simulink library "AEMS_Standard_Library"  (R2016b)
settings: Solver=ode45  StartTime=0.0  StopTime=10.0  RelTol=1e-3
undefined symbols (not defined in the file or in its folder): BkPY, carto, Cbx_extegr, Cbx_lpegrsys, Cbx_portegr, Cnx_bnk_nr_conf, Cnx_cyl_nr_conf, ConfigManagement, configuration_management, Cxx_dcm_io_tmr_end_xxxx, Cxx_dcm_rt_tmr_end, Cxx_DID_xxxx_IO_max, Cxx_DID_xxxx_IO_min, Cxx_egrhsofs, Cxx_vmaniegi, DEM_DEBOUNCE_FREEZE, DEM_DTR_CTL_INVISIBLE, DEM_DTR_CTL_NORMAL, Dem_DtrId2_XXX, Dem_DtrId3_XXX, Dem_DtrId4_XXX, Dem_DtrId5_XXX, Dem_DtrId6_XXX, Dem_DtrId7_XXX, Dem_DtrId8_XXX, Dem_DtrId9_XXX, Dem_DtrId_XXX, Dem_EnableConditionId2_XXX, Dem_EnableConditionId3_XXX, Dem_EnableConditionId4_XXX, Dem_EnableConditionId5_XXX, Dem_EnableConditionId6_XXX, Dem_EnableConditionId7_XXX, Dem_EnableConditionId8_XXX, Dem_EnableConditionId_XXX, Dem_EventId, Dem_EventId2_XXX, Dem_EventId3_XXX, Dem_EventId4_XXX, Dem_EventId5_XXX, Dem_EventId6_XXX, Dem_EventId7_XXX, Dem_EventId8_XXX, Dem_EventId9_XXX, Dem_EventId_Device_Faulttype, Dem_EventId_XXX, DEM_IUMPR_GENERAL_DENOMINATOR, DEM_OPCYC_IGNITION, Dem_RatioId2_XXX, Dem_RatioId3_XXX, Dem_RatioId4_XXX, Dem_RatioId5_XXX, Dem_RatioId6_XXX, Dem_RatioId7_XXX, Dem_RatioId8_XXX, Dem_RatioId_XXX, Dem_StorageConditionId2_XXX, Dem_StorageConditionId3_XXX, Dem_StorageConditionId4_XXX, Dem_StorageConditionId5_XXX ... (+65)
libraries: AEMS_Standard_Library x477, simulink x2
(part 18 of 39)

== system AEMS_Standard_Library/SPECIFIC/AEMS_AIR_BALANCE ==
  rpm : Inport  OutDataTypeStr=single  PortDimensions=1  Interpolate=off
  vcyl : Inport  Port=2  OutDataTypeStr=single  PortDimensions=1  Interpolate=off
  egclrt : Inport  Port=3  OutDataTypeStr=single  PortDimensions=1  Interpolate=off
  tanmnp : Inport  Port=4  OutDataTypeStr=single  PortDimensions=1  Interpolate=off
  fqselgo : Inport  Port=5  OutDataTypeStr=boolean  PortDimensions=1  Interpolate=off
  pargeqd : Inport  Port=6  OutDataTypeStr=single  PortDimensions=1  Interpolate=off
  qegrve : Inport  Port=7  OutDataTypeStr=single  PortDimensions=1  Interpolate=off
  ppamb : Inport  Port=8  OutDataTypeStr=single  PortDimensions=1  Interpolate=off
  qtrm : Inport  Port=9  OutDataTypeStr=single  PortDimensions=1  Interpolate=off
  qegrth : Inport  Port=10  OutDataTypeStr=single  PortDimensions=1  Interpolate=off
  fafmlmsta : Inport  Port=11  OutDataTypeStr=boolean  PortDimensions=1  Interpolate=off
  qcylegr_p : Inport  Port=12  OutDataTypeStr=single  PortDimensions=1  Interpolate=off
  vmani : Inport  Port=13  OutDataTypeStr=single  PortDimensions=1  Interpolate=off
  fair_egrv : Inport  Port=14  OutDataTypeStr=boolean  Interpolate=off
  MWI_Cyl_Charge_Mass_Air_N : Subsystem  Description=|
      | Air,EGR or (Air + EGR) mass of cylinder is calculated.                
      | Qcyl(kg/s)                                                            
      | = mamani(kg/1 cycle 1cylinder) * rpm * Nref(number of cylinder/2) * 60
  MWI_Mani_Charge_Mass_Air_EGR : Subsystem  Description=Air,EGR or (air+EGR) mass of correcter is calculated.
  MWI_Manifold_Pressure_N : Subsystem  Description=Pressure of correcter is calculated by the state equation.
  Unit Delay4 : UnitDelay  SampleTime=-1
      settings: AttributesFormatString=<initial=%<InitialCondition>>
  Unit Delay5 : UnitDelay  SampleTime=-1
      settings: AttributesFormatString=<initial=%<InitialCondition>>
  Unit Delay6 : UnitDelay  SampleTime=-1
      settings: AttributesFormatString=<initial=%<InitialCondition>>
  mamani : Outport
  airmani : Outport  Port=2
  macyllj : Outport  Port=3
  qcylall : Outport  Port=4
  qcylegr : Outport  Port=5
  qcyl : Outport  Port=6
  pmani : Outport  Port=7
  egrmani : Outport  Port=8
  egclrt_p : Outport  Port=9
  wires:
  vmani/1 -> MWI_Manifold_Pressure_N/1(vmani), MWI_Cyl_Charge_Mass_Air_N/5(vmani), MWI_Mani_Charge_Mass_Air_EGR/9(vmani)  "vmani"
  MWI_Cyl_Charge_Mass_Air_N/5(egclrt_p) -> egclrt_p/1
  qcylegr_p/1 -> MWI_Cyl_Charge_Mass_Air_N/4(qcylegr_p)  "qcylegr_p"
  fafmlmsta/1 -> MWI_Mani_Charge_Mass_Air_EGR/8(fafmlmsta)  "fafmlmsta"
  qegrth/1 -> MWI_Mani_Charge_Mass_Air_EGR/7(qegrth)  "qegrth"
  qtrm/1 -> MWI_Mani_Charge_Mass_Air_EGR/6(qtrm)  "qtrm"
  ppamb/1 -> MWI_Mani_Charge_Mass_Air_EGR/5(ppamb)  "ppamb"
  qegrve/1 -> MWI_Mani_Charge_Mass_Air_EGR/4(qegrve)  "qegrve"
  pargeqd/1 -> MWI_Mani_Charge_Mass_Air_EGR/3(pargeqd)  "pargeqd"
  fqselgo/1 -> MWI_Mani_Charge_Mass_Air_EGR/2(fqselgo)  "fqselgo"
  tanmnp/1 -> MWI_Manifold_Pressure_N/2(tanmnp), MWI_Mani_Charge_Mass_Air_EGR/1(tanmnp)  "tanmnp"
  egclrt/1 -> MWI_Cyl_Charge_Mass_Air_N/3(egclrt)  "egclrt"
  vcyl/1 -> MWI_Cyl_Charge_Mass_Air_N/2(vcyl)  "vcyl"
  rpm/1 -> MWI_Cyl_Charge_Mass_Air_N/1(rpm)  "rpm"
  MWI_Mani_Charge_Mass_Air_EGR/2(airmani) -> MWI_Manifold_Pressure_N/3(airmani), airmani/1
  MWI_Cyl_Charge_Mass_Air_N/4(macyllj) -> macyllj/1
  MWI_Manifold_Pressure_N/1(pmani) -> pmani/1
  Unit Delay6/1 -> MWI_Mani_Charge_Mass_Air_EGR/11(qcyl_pudt)  "qcyl_pudt"
  Unit Delay4/1 -> MWI_Mani_Charge_Mass_Air_EGR/12(qcylegr_pudt)  "qcylegr_pudt"
  Unit Delay5/1 -> MWI_Mani_Charge_Mass_Air_EGR/13(qcylall_pudt)  "qcylall_pudt"
  MWI_Mani_Charge_Mass_Air_EGR/3(egrmani) -> egrmani/1, MWI_Manifold_Pressure_N/4(egrmani)
  MWI_Mani_Charge_Mass_Air_EGR/1(mamani) -> MWI_Cyl_Charge_Mass_Air_N/6(mamani), mamani/1
  MWI_Cyl_Charge_Mass_Air_N/3(qcylall) -> qcylall/1, Unit Delay5/1
  MWI_Cyl_Charge_Mass_Air_N/2(qcylegr) -> qcylegr/1, Unit Delay4/1
  MWI_Cyl_Charge_Mass_Air_N/1(qcyl) -> Unit Delay6/1, qcyl/1
  fair_egrv/1 -> MWI_Mani_Charge_Mass_Air_EGR/10(fair_egrv)  "fair_egrv"

== system AEMS_Standard_Library/SPECIFIC/AEMS_AS_PADE ==
  Filter_param : Inport
  Vxx_in : Inport  Port=2
  Vxx_dly_t : Inport  Port=3
  Vbx_dly_init_ena : Inport  Port=4
  A_pade_model : Subsystem
  Saturation : Saturate  UpperLimit=2000  LowerLimit=0  RndMeth=Zero
      settings: AttributesFormatString=<limits=%<UpperLimit>/%<LowerLimit>>
  Vxx_in_dly : Outport
  Vxx_in_fil : Outport  Port=2
  wires:
  A_pade_model/1(Vxx_in_dly) -> Vxx_in_dly/1
  Vxx_in/1 -> A_pade_model/2(Vxx_in)
  Vbx_dly_init_ena/1 -> A_pade_model/4(Vbx_dly_init_ena)
  Vxx_dly_t/1 -> A_pade_model/3(Vxx_dly_t)
  A_pade_model/2(Vxx_in_fil) -> Saturation/1
  Saturation/1 -> Vxx_in_fil/1
  Filter_param/1 -> A_pade_model/1(Filter_param)

== system AEMS_Standard_Library/SPECIFIC/AEMS_AT_EHR ==
  Vxx_ehr_sel_tenv : Inport
  Vxx_ehr_sys_egaf : Inport  Port=2
  Vxx_ehr_cnvt_fac : Inport  Port=3
  Vxx_ehr_ext_exch_ar : Inport  Port=4
  Vxx_ehr_wht : Inport  Port=5
  Vxx_ehr_utp : Inport  Port=6
  Vxx_ehr_cata_temp_dly : Inport  Port=7
  Vxx_ehr_exo_pow : Inport  Port=8
  Vxx_ehr_spc_ex_gas_temp_cpy : Inport  Port=9
  Vxx_ehr_spc_cata_temp_cpy : Inport  Port=10
  Vxx_ehr_samp_t : Inport  Port=11
  A_Enabled_Calculation : Subsystem
  Vxx_ehr_dtp : Outport
  Vxx_ehr_ext_pow_loss : Outport  Port=2
  Vxx_ehr_wht_entr : Outport  Port=3
  Vxx_ehr_ex_gas_entr : Outport  Port=4
  Vxx_ehr_ext_cnvt_entr : Outport  Port=5
  Vxx_ehr_exo_temp_flu : Outport  Port=6
  Vxx_ehr_wht_temp_flu : Outport  Port=7
  Vxx_ehr_ex_gas_temp_flu : Outport  Port=8
  Vxx_ehr_ext_cnvt_temp_flu : Outport  Port=9
  wires:
  Vxx_ehr_sel_tenv/1 -> A_Enabled_Calculation/1(Vxx_ehr_sel_tenv)
  Vxx_ehr_cnvt_fac/1 -> A_Enabled_Calculation/2(Vxx_ehr_cnvt_fac)
  Vxx_ehr_ext_exch_ar/1 -> A_Enabled_Calculation/3(Vxx_ehr_ext_exch_ar)
  Vxx_ehr_samp_t/1 -> A_Enabled_Calculation/4(Vxx_ehr_samp_t)
  Vxx_ehr_utp/1 -> A_Enabled_Calculation/7(Vxx_ehr_utp)
  Vxx_ehr_sys_egaf/1 -> A_Enabled_Calculation/5(Vxx_ehr_sys_egaf)
  Vxx_ehr_spc_ex_gas_temp_cpy/1 -> A_Enabled_Calculation/10(Vxx_ehr_spc_ex_gas_temp_cpy)
  Vxx_ehr_spc_cata_temp_cpy/1 -> A_Enabled_Calculation/11(Vxx_ehr_spc_cata_temp_cpy)
  Vxx_ehr_cata_temp_dly/1 -> A_Enabled_Calculation/8(Vxx_ehr_cata_temp_dly)
  Vxx_ehr_exo_pow/1 -> A_Enabled_Calculation/9(Vxx_ehr_exo_pow)
  Vxx_ehr_wht/1 -> A_Enabled_Calculation/6(Vxx_ehr_wht)
  A_Enabled_Calculation/1(Vxx_ehr_dtp) -> Vxx_ehr_dtp/1
  A_Enabled_Calculation/2(Vxx_ehr_ext_pow_loss) -> Vxx_ehr_ext_pow_loss/1
  A_Enabled_Calculation/3(Vxx_ehr_wht_entr) -> Vxx_ehr_wht_entr/1
  A_Enabled_Calculation/4(Vxx_ehr_ex_gas_entr) -> Vxx_ehr_ex_gas_entr/1
  A_Enabled_Calculation/5(Vxx_ehr_ext_cnvt_entr) -> Vxx_ehr_ext_cnvt_entr/1
  A_Enabled_Calculation/6(Vxx_ehr_exo_temp_flu) -> Vxx_ehr_exo_temp_flu/1
  A_Enabled_Calculation/7(Vxx_ehr_wht_temp_flu) -> Vxx_ehr_wht_temp_flu/1
  A_Enabled_Calculation/8(Vxx_ehr_ex_gas_temp_flu) -> Vxx_ehr_ex_gas_temp_flu/1
  A_Enabled_Calculation/9(Vxx_ehr_ext_cnvt_temp_flu) -> Vxx_ehr_ext_cnvt_temp_flu/1

== system AEMS_Standard_Library/SPECIFIC/AEMS_AT_TUBE ==
  Vxx_tub_utp : Inport
  Vxx_tub_utp_dly : Inport  Port=2
  Vxx_tub_egaf : Inport  Port=3
  Vxx_tub_temp_air : Inport  Port=4
  Vxx_tub_pow_ext : Inport  Port=5
  Vxx_tub_itl_ar : Inport  Port=6
  Vxx_tub_itl_cnvt_fac : Inport  Port=7
  Vxx_tub_ext_ar : Inport  Port=8
  Vxx_tub_ext_cnvt_fac : Inport  Port=9
  Vxx_tub_wht : Inport  Port=10
  Vxx_tub_temp_rd_loss : Inport  Port=11
  Vxx_tub_itl_gas_wht_cor : Inport  Port=12
  Vxx_tub_cal_cpy : Inport  Port=13
  Vxx_tub_gas_cal_cpy : Inport  Port=14
  Vxx_tub_utp_gas_wht_cor : Inport  Port=15
  Vxx_tub_samp_t : Inport  Port=16
  Vxx_tub_temp_esti_dly : Inport  Port=17
  Vxx_tub_ex_gas_dtp_esti_dly : Inport  Port=18
  A_Thermal_Calculation : Subsystem
  Vxx_tub_ex_gas_dtp_esti : Outport
  Vxx_tub_temp_esti : Outport  Port=2
  Vxx_tub_ex_gas_pow_loss : Outport  Port=3
  Vxx_tub_temp_pow_loss : Outport  Port=4
  Vxx_tub_temp_rd_entr : Outport  Port=5
  Vxx_tub_wht_entr : Outport  Port=6
  Vxx_tub_itl_cnvt_entr : Outport  Port=7
  Vxx_tub_ext_cnvt_entr : Outport  Port=8
  Vxx_tub_entr_tot : Outport  Port=9
  Vxx_tub_ext_cnvt_temp_flu : Outport  Port=10
  Vxx_tub_itl_cnvt_temp_flu : Outport  Port=11
  Vxx_tub_wht_temp_flu : Outport  Port=12
  Vxx_tub_ex_gas_entr : Outport  Port=13
  Vxx_tub_itl_gas_wht_entr : Outport  Port=14
  Vxx_tub_itl_gas_cnvt_entr : Outport  Port=15
  Vxx_tub_gas_entr_tot : Outport  Port=16
  Vxx_tub_gas_temp_flu : Outport  Port=17
  Vxx_tub_gas_wht_temp_flu : Outport  Port=18
  Vxx_tub_gas_itl_cnvt_temp_flu : Outport  Port=19
  Vxx_tub_gas_utp_wht_temp_flu : Outport  Port=20
  Vxx_tub_gas_ext_egy_temp_flu : Outport  Port=21
  wires:
  A_Thermal_Calculation/21(Vxx_tub_gas_ext_egy_temp_flu) -> Vxx_tub_gas_ext_egy_temp_flu/1
  A_Thermal_Calculation/20(Vxx_tub_gas_utp_wht_temp_flu) -> Vxx_tub_gas_utp_wht_temp_flu/1
  A_Thermal_Calculation/19(Vxx_tub_gas_itl_cnvt_temp_flu) -> Vxx_tub_gas_itl_cnvt_temp_flu/1
  A_Thermal_Calculation/18(Vxx_tub_gas_wht_temp_flu) -> Vxx_tub_gas_wht_temp_flu/1
  A_Thermal_Calculation/17(Vxx_tub_gas_temp_flu) -> Vxx_tub_gas_temp_flu/1
  A_Thermal_Calculation/16(Vxx_tub_gas_entr_tot) -> Vxx_tub_gas_entr_tot/1
  A_Thermal_Calculation/15(Vxx_tub_itl_gas_cnvt_entr) -> Vxx_tub_itl_gas_cnvt_entr/1
  A_Thermal_Calculation/14(Vxx_tub_itl_gas_wht_entr) -> Vxx_tub_itl_gas_wht_entr/1
  A_Thermal_Calculation/13(Vxx_tub_ex_gas_entr) -> Vxx_tub_ex_gas_entr/1
  A_Thermal_Calculation/12(Vxx_tub_wht_temp_flu) -> Vxx_tub_wht_temp_flu/1
  A_Thermal_Calculation/11(Vxx_tub_itl_cnvt_temp_flu) -> Vxx_tub_itl_cnvt_temp_flu/1
  A_Thermal_Calculation/10(Vxx_tub_ext_cnvt_temp_flu) -> Vxx_tub_ext_cnvt_temp_flu/1
  A_Thermal_Calculation/9(Vxx_tub_entr_tot) -> Vxx_tub_entr_tot/1
  A_Thermal_Calculation/8(Vxx_tub_ext_cnvt_entr) -> Vxx_tub_ext_cnvt_entr/1
  A_Thermal_Calculation/7(Vxx_tub_itl_cnvt_entr) -> Vxx_tub_itl_cnvt_entr/1
  A_Thermal_Calculation/6(Vxx_tub_wht_entr) -> Vxx_tub_wht_entr/1
  A_Thermal_Calculation/5(Vxx_tub_temp_rd_entr) -> Vxx_tub_temp_rd_entr/1
  A_Thermal_Calculation/4(Vxx_tub_temp_pow_loss) -> Vxx_tub_temp_pow_loss/1
  A_Thermal_Calculation/3(Vxx_tub_ex_gas_pow_loss) -> Vxx_tub_ex_gas_pow_loss/1
  A_Thermal_Calculation/2(Vxx_tub_temp_esti) -> Vxx_tub_temp_esti/1
  A_Thermal_Calculation/1(Vxx_tub_ex_gas_dtp_esti) -> Vxx_tub_ex_gas_dtp_esti/1
  Vxx_tub_ex_gas_dtp_esti_dly/1 -> A_Thermal_Calculation/18(Vxx_tub_ex_gas_dtp_esti_dly)
  Vxx_tub_temp_esti_dly/1 -> A_Thermal_Calculation/17(Vxx_tub_temp_esti_dly)
  Vxx_tub_samp_t/1 -> A_Thermal_Calculation/16(Vxx_tub_samp_t)
  Vxx_tub_utp_gas_wht_cor/1 -> A_Thermal_Calculation/15(Vxx_tub_utp_gas_wht_cor)
  Vxx_tub_gas_cal_cpy/1 -> A_Thermal_Calculation/14(Vxx_tub_gas_cal_cpy)
  Vxx_tub_cal_cpy/1 -> A_Thermal_Calculation/13(Vxx_tub_cal_cpy)
  Vxx_tub_itl_gas_wht_cor/1 -> A_Thermal_Calculation/12(Vxx_tub_itl_gas_wht_cor)
  Vxx_tub_temp_rd_loss/1 -> A_Thermal_Calculation/11(Vxx_tub_temp_rd_loss)
  Vxx_tub_wht/1 -> A_Thermal_Calculation/10(Vxx_tub_wht)
  Vxx_tub_ext_cnvt_fac/1 -> A_Thermal_Calculation/9(Vxx_tub_ext_cnvt_fac)
  Vxx_tub_ext_ar/1 -> A_Thermal_Calculation/8(Vxx_tub_ext_ar)
  Vxx_tub_itl_cnvt_fac/1 -> A_Thermal_Calculation/7(Vxx_tub_itl_cnvt_fac)
  Vxx_tub_itl_ar/1 -> A_Thermal_Calculation/6(Vxx_tub_itl_ar)
  Vxx_tub_pow_ext/1 -> A_Thermal_Calculation/5(Vxx_tub_pow_ext)
  Vxx_tub_temp_air/1 -> A_Thermal_Calculation/4(Vxx_tub_temp_air)
  Vxx_tub_egaf/1 -> A_Thermal_Calculation/3(Vxx_tub_egaf)
  Vxx_tub_utp_dly/1 -> A_Thermal_Calculation/2(Vxx_tub_utp_dly)
  Vxx_tub_utp/1 -> A_Thermal_Calculation/1(Vxx_tub_utp)

== system AEMS_Standard_Library/SPECIFIC/AEMS_BACKUP_FOR_ENGINE_OFF_MONITOR ==
  set : Inport  OutDataTypeStr=boolean
  AND : Logic  OutDataTypeStr=boolean
  AND1 : Logic  Operator=OR  OutDataTypeStr=boolean
  Unit Delay : UnitDelay  SampleTime=-1
      settings: AttributesFormatString=<initial=%<InitialCondition>>
  Unit Delay1 : UnitDelay  SampleTime=-1
      settings: AttributesFormatString=<initial=%<InitialCondition>>
  one : Constant  OutDataTypeStr=boolean
  flag : Outport
  wires:
  Unit Delay/1 -> AND/2
  AND1/1 -> flag/1, Unit Delay/1  "flag"
  set/1 -> AND1/1  "set"
  AND/1 -> AND1/2
  one/1 -> Unit Delay1/1  "one"
  Unit Delay1/1 -> AND/1

== system AEMS_Standard_Library/SPECIFIC/AEMS_BACK_UP ==
  start_flag : Inport
      settings: AttributesFormatString=<tsample=%<sampleTime>>
  vback_up_variable : Inport  Port=2
      settings: AttributesFormatString=<tsample=%<sampleTime>>
  MinMax1 : MinMax  Function=max  Inputs=2  SaturateOnIntegerOverflow=on  InputSameDT=on
  MinMax3 : MinMax  Inputs=2  SaturateOnIntegerOverflow=on  InputSameDT=on
  Switch1 : Switch  Criteria=u2 ~= 0  InputSameDT=on
      settings: AttributesFormatString=Criteria=%<Criteria>
  Switch2 : Switch  Criteria=u2 ~= 0  InputSameDT=on
      settings: AttributesFormatString=Criteria=%<Criteria>
  Switch4 : Switch  Criteria=u2 ~= 0  InputSameDT=on
      settings: AttributesFormatString=Criteria=%<Criteria>
  Unit Delay : UnitDelay  InitialCondition=max_parameter  SampleTime=-1
      settings: AttributesFormatString=<initial=%<InitialCondition>>
  Unit Delay1 : UnitDelay  InitialCondition=min_parameter  SampleTime=-1
      settings: AttributesFormatString=<initial=%<InitialCondition>>
  Unit Delay3 : UnitDelay  SampleTime=-1
      settings: AttributesFormatString=<initial=%<InitialCondition>>
  vend_value : Outport
  vmin_value : Outport  Port=2
  vmax_value : Outport  Port=3
  wires:
  vback_up_variable/1 -> Switch4/1, MinMax3/1, MinMax1/1  "vback_up_variable"
  Switch1/1 -> Unit Delay/1, vmin_value/1  "vmin_value"
  Unit Delay/1 -> MinMax3/2, Switch1/3
  MinMax3/1 -> Switch1/1
  Switch2/1 -> Unit Delay1/1, vmax_value/1  "vmax_value"
  Unit Delay1/1 -> MinMax1/2, Switch2/3
  MinMax1/1 -> Switch2/1
  start_flag/1 -> Switch4/2, Switch1/2, Switch2/2  "start_flag"
  Unit Delay3/1 -> Switch4/3
  Switch4/1 -> Unit Delay3/1, vend_value/1  "vend_value"

== system AEMS_Standard_Library/SPECIFIC/AEMS_BACK_UP_AVE ==
  start_flag : Inport
      settings: AttributesFormatString=<tsample=%<sampleTime>>
  vback_up_variable : Inport  Port=2
      settings: AttributesFormatString=<tsample=%<sampleTime>>
  AEMS_COUNTER : AEMS_Standard_Library/COUNTER/AEMS_COUNTER  Tag=[LIB]  mMAX=2byte
      settings: AttributesFormatString=%<MaskType>\nMax. count range = %<mMAX>
  MinMax1 : MinMax  Function=max  Inputs=2  SaturateOnIntegerOverflow=on  InputSameDT=on
  MinMax2 : MinMax  Function=max  Inputs=2  SaturateOnIntegerOverflow=on  InputSameDT=on
  MinMax3 : MinMax  Inputs=2  SaturateOnIntegerOverflow=on  InputSameDT=on
  MinMax5 : MinMax  Function=max  Inputs=2  SaturateOnIntegerOverflow=on  InputSameDT=on
  MinMax6 : MinMax  Inputs=2  SaturateOnIntegerOverflow=on  InputSameDT=on
  Product1 : Product  Inputs=**  OutDataTypeStr=Inherit: Inherit via back propagation  SaturateOnIntegerOverflow=on  RndMeth=Zero
      settings: AttributesFormatString=SAT = %<SaturateOnIntegerOverflow>
  Product3 : Product  Inputs=*/  OutDataTypeStr=Inherit: Inherit via back propagation  RndMeth=Zero
  Product4 : Product  Inputs=**  OutDataTypeStr=Inherit: Inherit via back propagation  SaturateOnIntegerOverflow=on  RndMeth=Zero
      settings: AttributesFormatString=SAT = %<SaturateOnIntegerOverflow>
  Sum1 : Sum  SaturateOnIntegerOverflow=on  InputSameDT=on  OutDataTypeStr=Inherit: Same as first input
  Switch{1..5} (5 alike) : Switch  Criteria=u2 ~= 0  InputSameDT=on
      settings: AttributesFormatString=Criteria=%<Criteria>
  Unit Delay : UnitDelay  InitialCondition=max_parameter  SampleTime=-1
      settings: AttributesFormatString=<initial=%<InitialCondition>>
  Unit Delay1 : UnitDelay  InitialCondition=min_parameter  SampleTime=-1
      settings: AttributesFormatString=<initial=%<InitialCondition>>
  Unit Delay2 : UnitDelay  SampleTime=-1
      settings: AttributesFormatString=<initial=%<InitialCondition>>
  Unit Delay3 : UnitDelay  SampleTime=-1
      settings: AttributesFormatString=<initial=%<InitialCondition>>
  Unit Delay4 : UnitDelay  SampleTime=-1
      settings: AttributesFormatString=<initial=%<InitialCondition>>
  imm_const1 : Constant  OutDataTypeStr=Inherit: Inherit via back propagation
  imm_const2 : Constant  Value=min_parameter  OutDataTypeStr=Inherit: Inherit via back propagation
  imm_const3 : Constant  Value=0  OutDataTypeStr=boolean
  imm_const5 : Constant  Value=65535  OutDataTypeStr=Inherit: Inherit via back propagation
  imm_const6 : Constant  Value=max_parameter  OutDataTypeStr=Inherit: Inherit via back propagation
  vend_value : Outport
  vmin_value : Outport  Port=2
  vmax_value : Outport  Port=3
  vaverage_value : Outport  Port=4
  wires:
  MinMax1/1 -> Switch2/1
  Unit Delay3/1 -> Switch4/3
  Switch4/1 -> vend_value/1, Unit Delay3/1  "vend_value"
  imm_const2/1 -> Product1/1
  imm_const6/1 -> Product4/1
  imm_const5/1 -> Product4/2, Product1/2  "vmax_count"
  Switch5/1 -> vaverage_value/1, Unit Delay4/1  "vaverage_value"
  Unit Delay4/1 -> Switch5/3
  imm_const3/1 -> AEMS_COUNTER/2  "clear"
  Sum1/1 -> MinMax6/1  "vsum_value"
  Product1/1 -> MinMax5/2
  MinMax6/1 -> MinMax5/1
  MinMax5/1 -> Switch3/1
  Product4/1 -> MinMax6/2
  Product3/1 -> Switch5/1  "average"
  start_flag/1 -> Switch3/2, AEMS_COUNTER/1, Switch5/2, Switch2/2, Switch1/2, Switch4/2
  Switch3/1 -> Unit Delay2/1, Product3/1  "vsum_value"
  imm_const1/1 -> MinMax2/1
  MinMax2/1 -> Product3/2
  Unit Delay2/1 -> Sum1/2, Switch3/3
  AEMS_COUNTER/1 -> MinMax2/2
  vback_up_variable/1 -> MinMax3/1, Sum1/1, MinMax1/1, Switch4/1
  Unit Delay1/1 -> Switch2/3, MinMax1/2
  MinMax3/1 -> Switch1/1
  Unit Delay/1 -> Switch1/3, MinMax3/2
  Switch2/1 -> vmax_value/1, Unit Delay1/1  "vmax_value"
  Switch1/1 -> vmin_value/1, Unit Delay/1  "vmin_value"

== system AEMS_Standard_Library/SPECIFIC/AEMS_DGNDMDPGCUT ==
  note: DGNDMDPGCUT
  mpr : Inport
  dgndmdpc : Inport  Port=2
  kdutydgn : Inport  Port=3
  mxmprp : Inport  Port=4
  AEMS_EDGE_RISING : AEMS_Standard_Library/EDGE/AEMS_EDGE_RISING  Tag=[LIB]  init=false
      settings: AttributesFormatString=|
      | %<MaskType>
      | Initial Value : %<init>
  Product1 : Product  OutDataTypeStr=Inherit: Inherit via back propagation  RndMeth=Zero
  Switch : Switch  Criteria=u2 ~= 0  SaturateOnIntegerOverflow=on  InputSameDT=on
      settings: AttributesFormatString=Criteria=%<Criteria>
  Switch1 : Switch  Criteria=u2 ~= 0  SaturateOnIntegerOverflow=on  InputSameDT=on
      settings: AttributesFormatString=Criteria=%<Criteria>
  Unit Delay3 : UnitDelay  SampleTime=-1
      settings: AttributesFormatString=<initial=%<InitialCondition>>
  mprmax : Outport
  wires:
  Product1/1 -> Switch1/1
  dgndmdpc/1 -> Switch1/2, AEMS_EDGE_RISING/1
  kdutydgn/1 -> Product1/1
  mxmprp/1 -> Switch1/3
  Switch/1 -> Product1/2, Unit Delay3/1  "tmp"
  AEMS_EDGE_RISING/1 -> Switch/2
  mpr/1 -> Switch/1
  Unit Delay3/1 -> Switch/3
  Switch1/1 -> mprmax/1  "mprmax"

== system AEMS_Standard_Library/SPECIFIC/AEMS_DGN_BB_RESULT ==
  fdgn_dgnsw : Inport  OutDataTypeStr=boolean  Interpolate=off
  dataclr : Inport  Port=2  OutDataTypeStr=boolean  Interpolate=off
  fdgn_raw : Inport  Port=3  OutDataTypeStr=boolean  PortDimensions=1  Interpolate=off
  fdgn_avl : Inport  Port=4  OutDataTypeStr=boolean  Interpolate=off
  fdgn_fs : Inport  Port=5  OutDataTypeStr=boolean
  fdgn_nbc : Inport  Port=6  OutDataTypeStr=boolean
  mdgn_ngt : Inport  Port=7  Interpolate=off
  mdgn_ngc : Inport  Port=8  Interpolate=off
  mdgn_hc : Inport  Port=9  Interpolate=off
  DGN_BB_Result_Counter : Subsystem
  vdgn_okcnt : Outport
  vdgn_cnt : Outport  Port=2
  fdgn_fsok : Outport  Port=3
  fdgn_dgntrp : Outport  Port=4
  fdgn_dgnok : Outport  Port=5
  wires:
  dataclr/1 -> DGN_BB_Result_Counter/1(dataclr)  "dataclr"
  fdgn_raw/1 -> DGN_BB_Result_Counter/2(fdgn_raw)  "fdgn_raw"
  fdgn_fs/1 -> DGN_BB_Result_Counter/3(fdgn_fs)  "fdgn_fs"
  fdgn_nbc/1 -> DGN_BB_Result_Counter/4(fdgn_nbc)  "fdgn_nbc"
  mdgn_ngt/1 -> DGN_BB_Result_Counter/5(mdgn_ngt)  "mdgn_ngt"
  mdgn_ngc/1 -> DGN_BB_Result_Counter/6(mdgn_ngc)  "mdgn_ngc"
  mdgn_hc/1 -> DGN_BB_Result_Counter/7(mdgn_hc)  "mdgn_hc"
  fdgn_avl/1 -> DGN_BB_Result_Counter/8(fdgn_avl)  "fdgn_avl"
  fdgn_dgnsw/1 -> DGN_BB_Result_Counter/Enable  "fdgn_dgnsw"
  DGN_BB_Result_Counter/1(vdgn_okcnt) -> vdgn_okcnt/1
  DGN_BB_Result_Counter/2(vdgn_cnt) -> vdgn_cnt/1
  DGN_BB_Result_Counter/3(fdgn_fsok) -> fdgn_fsok/1
  DGN_BB_Result_Counter/4(fdgn_dgntrp) -> fdgn_dgntrp/1
  DGN_BB_Result_Counter/5(fdgn_dgnok) -> fdgn_dgnok/1

== system AEMS_Standard_Library/SPECIFIC/AEMS_DGN_MF_MISX_CALCULATION_LIB ==
  vtint_den_mem : Inport
  vtint_num_mem : Inport  Port=2
  index_base : Inport  Port=3
  index_pre : Inport  Port=4
  index_post : Inport  Port=5
  index_den : Inport  Port=6
  vtint_pre_times : Inport  Port=7
  vtint_post_times : Inport  Port=8
  mmsu : Inport  Port=9
  vtp : Inport  Port=10
  vmisxhos : Inport  Port=11
  DGN_MF_misx_calcuration_lib_AEMS : Stateflow chart
  vmisx : Outport
  wires:
  vmisxhos/1 -> DGN_MF_misx_calcuration_lib_AEMS/11(vmisxhos)
  vtint_den_mem/1 -> DGN_MF_misx_calcuration_lib_AEMS/1(vtint_den_mem)
  vtp/1 -> DGN_MF_misx_calcuration_lib_AEMS/10(vtp)
  mmsu/1 -> DGN_MF_misx_calcuration_lib_AEMS/9(mmsu)
  vtint_post_times/1 -> DGN_MF_misx_calcuration_lib_AEMS/8(vtint_post_times)
  vtint_pre_times/1 -> DGN_MF_misx_calcuration_lib_AEMS/7(vtint_pre_times)
  index_post/1 -> DGN_MF_misx_calcuration_lib_AEMS/5(index_post)
  vtint_num_mem/1 -> DGN_MF_misx_calcuration_lib_AEMS/2(vtint_num_mem)
  index_den/1 -> DGN_MF_misx_calcuration_lib_AEMS/6(index_den)
  index_base/1 -> DGN_MF_misx_calcuration_lib_AEMS/3(index_base)
  index_pre/1 -> DGN_MF_misx_calcuration_lib_AEMS/4(index_pre)
  DGN_MF_misx_calcuration_lib_AEMS/1(vmisx) -> vmisx/1

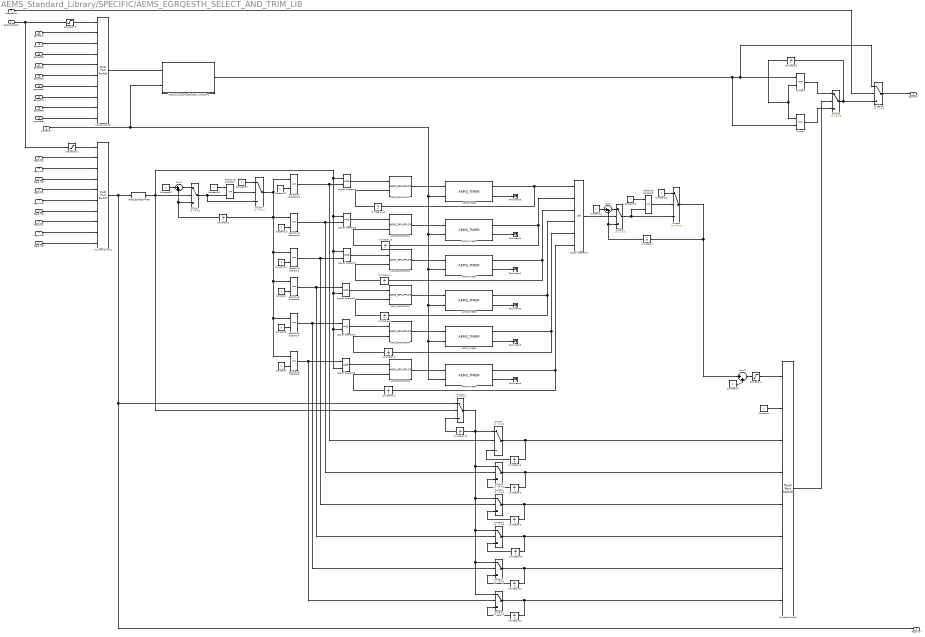
== system AEMS_Standard_Library/SPECIFIC/AEMS_EGRQESTH_SELECT_AND_TRIM_LIB ==
  egrtgstdly : Inport  OutDataTypeStr=single  PortDimensions=1
      settings: AttributesFormatString=<tsample=%<SampleTime>>
  egrblockselect : Inport  Port=2  OutDataTypeStr=single  PortDimensions=1
      settings: AttributesFormatString=<tsample=%<SampleTime>>
  fegrqinc9 : Inport  Port=3  OutDataTypeStr=boolean  PortDimensions=1
      settings: AttributesFormatString=<tsample=%<SampleTime>>
  fegrqinc8 : Inport  Port=4  OutDataTypeStr=boolean  PortDimensions=1
      settings: AttributesFormatString=<tsample=%<SampleTime>>
  fegrqinc7 : Inport  Port=5  OutDataTypeStr=boolean  PortDimensions=1
      settings: AttributesFormatString=<tsample=%<SampleTime>>
  fegrqinc6 : Inport  Port=6  OutDataTypeStr=boolean  PortDimensions=1
      settings: AttributesFormatString=<tsample=%<SampleTime>>
  fegrqinc5 : Inport  Port=7  OutDataTypeStr=boolean  PortDimensions=1
      settings: AttributesFormatString=<tsample=%<SampleTime>>
  fegrqinc4 : Inport  Port=8  OutDataTypeStr=boolean  PortDimensions=1
      settings: AttributesFormatString=<tsample=%<SampleTime>>
  fegrqinc3 : Inport  Port=9  OutDataTypeStr=boolean  PortDimensions=1
      settings: AttributesFormatString=<tsample=%<SampleTime>>
  fegrqinc2 : Inport  Port=10  OutDataTypeStr=boolean  PortDimensions=1
      settings: AttributesFormatString=<tsample=%<SampleTime>>
  fegrqinc1 : Inport  Port=11  OutDataTypeStr=boolean  PortDimensions=1
      settings: AttributesFormatString=<tsample=%<SampleTime>>
  egrqest9h : Inport  Port=12  OutDataTypeStr=single  PortDimensions=1
      settings: AttributesFormatString=<tsample=%<SampleTime>>
  egrqest8h : Inport  Port=13  OutDataTypeStr=single  PortDimensions=1
      settings: AttributesFormatString=<tsample=%<SampleTime>>
  egrqest7h : Inport  Port=14  OutDataTypeStr=single  PortDimensions=1
      settings: AttributesFormatString=<tsample=%<SampleTime>>
  egrqest6h : Inport  Port=15  OutDataTypeStr=single  PortDimensions=1
      settings: AttributesFormatString=<tsample=%<SampleTime>>
  egrqest5h : Inport  Port=16  OutDataTypeStr=single  PortDimensions=1
      settings: AttributesFormatString=<tsample=%<SampleTime>>
  egrqest4h : Inport  Port=17  OutDataTypeStr=single  PortDimensions=1
      settings: AttributesFormatString=<tsample=%<SampleTime>>
  egrqest3h : Inport  Port=18  OutDataTypeStr=single  PortDimensions=1
      settings: AttributesFormatString=<tsample=%<SampleTime>>
  egrqest2h : Inport  Port=19  OutDataTypeStr=single  PortDimensions=1
      settings: AttributesFormatString=<tsample=%<SampleTime>>
  egrqest1h : Inport  Port=20  OutDataTypeStr=single  PortDimensions=1
      settings: AttributesFormatString=<tsample=%<SampleTime>>
  mfegrcohsw : Inport  Port=21  OutDataTypeStr=boolean  PortDimensions=1
      settings: AttributesFormatString=<tsample=%<SampleTime>>
  AEMS_EDGE_EITHER : AEMS_Standard_Library/EDGE/AEMS_EDGE_EITHER  Tag=[LIB]  init=false
      settings: AttributesFormatString=|
      | %<MaskType>
      | Initial Value : %<init>
  AEMS_SRFLIPFLOP{,1..5} (6 alike) : AEMS_Standard_Library/FLAG/AEMS_SRFLIPFLOP  Tag=[LIB]  init=false
      settings: AttributesFormatString=%<MaskType>\nInitial condition (state of Q): = %<init>
  AEMS_TIMER{,1..5} (6 alike) : AEMS_Standard_Library/TIMER/AEMS_TIMER  Tag=[LIB]  sample_time=0.01
      settings: AttributesFormatString=%<MaskType>
  Constant1 : Constant  OutDataTypeStr=boolean
  Constant{11,13..14,22,29,33} (6 alike) : Constant  OutDataTypeStr=uint8
  Constant12 : Constant  Value=7  OutDataTypeStr=uint8
  Constant2 : Constant  Value=4  OutDataTypeStr=uint8
  Constant23 : Constant  Value=2  OutDataTypeStr=uint8
  Constant24 : Constant  Value=3  OutDataTypeStr=uint8
  Constant28 : Constant  Value=7  OutDataTypeStr=uint8
  Constant3 : Constant  Value=5  OutDataTypeStr=uint8
  Constant4 : Constant  Value=6  OutDataTypeStr=uint8
  Logical Operator1 : Logic  Operator=OR  Inputs=6  OutDataTypeStr=boolean
  Logical Operator{2..7} (6 alike) : Logic  OutDataTypeStr=boolean
  M2002_2A_2A_0x_EGR_DELAY_NR_10ms : Stateflow chart
  MinMax : MinMax  Inputs=2  SaturateOnIntegerOverflow=on  InputSameDT=on
  MinMax1 : MinMax  Function=max  Inputs=2  SaturateOnIntegerOverflow=on  InputSameDT=on
  Multiport Switch : MultiPortSwitch  Inputs=9  SaturateOnIntegerOverflow=on  InputSameDT=on
  Multiport Switch1 : MultiPortSwitch  Inputs=9  SaturateOnIntegerOverflow=on  InputSameDT=on
  Multiport Switch2 : MultiPortSwitch  Inputs=7  SaturateOnIntegerOverflow=on  InputSameDT=on
  Relational Operator{1,3..5,10,14} (6 alike) : RelationalOperator  Operator===  OutDataTypeStr=boolean  RndMeth=Nearest  InputSameDT=on
  Relational Operator2 : RelationalOperator  Operator=<=  OutDataTypeStr=boolean  RndMeth=Nearest  InputSameDT=on
  Relational Operator7 : RelationalOperator  Operator=<=  OutDataTypeStr=boolean  RndMeth=Nearest  InputSameDT=on
  Saturation1 : Saturate  UpperLimit=7  LowerLimit=1
      settings: AttributesFormatString=<limits=%<UpperLimit>/%<LowerLimit>>
  Saturation2 : Saturate  UpperLimit=9  LowerLimit=1
      settings: AttributesFormatString=<limits=%<UpperLimit>/%<LowerLimit>>
  Saturation3 : Saturate  UpperLimit=9  LowerLimit=1
      settings: AttributesFormatString=<limits=%<UpperLimit>/%<LowerLimit>>
  Sum : Sum  Inputs=|++  SaturateOnIntegerOverflow=on
  Sum2 : Sum  Inputs=|++  SaturateOnIntegerOverflow=on
  Sum3 : Sum  Inputs=|++  SaturateOnIntegerOverflow=on
  Switch{1..13} (13 alike) : Switch  Threshold=0.5  SaturateOnIntegerOverflow=on  InputSameDT=on
      Switch1 settings: AttributesFormatString=<threshold=%<threshold>>
      Switch10 settings: AttributesFormatString=<threshold=%<threshold>>
      Switch11 settings: AttributesFormatString=<threshold=%<threshold>>
      Switch12 settings: AttributesFormatString=<threshold=%<threshold>>
      Switch13 settings: AttributesFormatString=<Threshold=%<Threshold>>
      Switch2 settings: AttributesFormatString=<threshold=%<threshold>>
      Switch3 settings: AttributesFormatString=<threshold=%<threshold>>
      Switch4 settings: AttributesFormatString=<threshold=%<threshold>>
      Switch5 settings: AttributesFormatString=<threshold=%<threshold>>
      Switch6 settings: AttributesFormatString=<threshold=%<threshold>>
      Switch7 settings: AttributesFormatString=<threshold=%<threshold>>
      Switch8 settings: AttributesFormatString=<threshold=%<threshold>>
      Switch9 settings: AttributesFormatString=<Threshold=%<Threshold>>
  Terminator{1..6} (6 alike) : Terminator
  Unit Delay{1..5,7,11..13} (9 alike) : UnitDelay  SampleTime=-1
      settings: AttributesFormatString=<initial=%<X0>>
  Unit Delay{6,8..10,14..16} (7 alike) : UnitDelay  InitialCondition=1  SampleTime=-1
      settings: AttributesFormatString=<initial=%<X0>>
  fegrqincx : Outport
  egrqcoh : Outport  Port=2
  wires:
  Unit Delay13/1 -> AEMS_SRFLIPFLOP/2  "clear"
  Unit Delay12/1 -> AEMS_SRFLIPFLOP1/2  "clear"
  Unit Delay4/1 -> AEMS_SRFLIPFLOP2/2  "clear"
  Unit Delay5/1 -> AEMS_SRFLIPFLOP4/2  "clear"
  Unit Delay2/1 -> AEMS_SRFLIPFLOP3/2  "clear"
  Unit Delay11/1 -> AEMS_SRFLIPFLOP5/2  "clear"
  mfegrcohsw/1 -> Switch13/2  "mfegrcohsw"
  Switch13/1 -> egrqcoh/1  "egrqcoh"
  Unit Delay16/1 -> Switch12/3
  Switch12/1 -> Unit Delay16/1, Multiport Switch2/8  "temp"
  Unit Delay15/1 -> Switch11/3
  Switch11/1 -> Unit Delay15/1, Multiport Switch2/7  "temp"
  Unit Delay14/1 -> Switch10/3
  Switch10/1 -> Unit Delay14/1, Multiport Switch2/6  "temp"
  Logical Operator5/1 -> AEMS_SRFLIPFLOP5/1  "set"
  Relational Operator5/1 -> Logical Operator5/1, Switch12/2  "and6"
  Constant4/1 -> Relational Operator5/2
  Logical Operator3/1 -> AEMS_SRFLIPFLOP4/1  "set"
  Relational Operator4/1 -> Logical Operator3/1, Switch11/2  "and5"
  Constant3/1 -> Relational Operator4/2
  Logical Operator2/1 -> AEMS_SRFLIPFLOP3/1  "set"
  Relational Operator3/1 -> Logical Operator2/1, Switch10/2  "and4"
  Constant2/1 -> Relational Operator3/2
  AEMS_SRFLIPFLOP5/1 -> AEMS_TIMER5/1  "start_flag"
  AEMS_TIMER5/2 -> Terminator6/1
  AEMS_TIMER5/1 -> Unit Delay11/1, Logical Operator1/6  "clear"
  AEMS_SRFLIPFLOP4/1 -> AEMS_TIMER4/1  "start_flag"
  AEMS_TIMER4/2 -> Terminator5/1
  AEMS_TIMER4/1 -> Unit Delay5/1, Logical Operator1/5
  AEMS_SRFLIPFLOP3/1 -> AEMS_TIMER3/1  "start_flag"
  AEMS_TIMER3/2 -> Terminator2/1
  AEMS_TIMER3/1 -> Unit Delay2/1, Logical Operator1/4
  egrqest8h/1 -> Multiport Switch/9  "egrqest8h"
  egrqest7h/1 -> Multiport Switch/8  "egrqest7h"
  egrqest6h/1 -> Multiport Switch/7  "egrqest6h"
  egrqest5h/1 -> Multiport Switch/6  "egrqest5h"
  egrqest4h/1 -> Multiport Switch/5  "egrqest4h"
  egrqest3h/1 -> Multiport Switch/4  "egrqest3h"
  egrqest2h/1 -> Multiport Switch/3  "egrqest2h"
  egrqest1h/1 -> Multiport Switch/2  "egrqest1h"
  egrqest9h/1 -> Multiport Switch/10  "egrqest9h"
  egrblockselect/1 -> Saturation2/1, Saturation3/1  "egrblockselect"
  M2002_2A_2A_0x_EGR_DELAY_NR_10ms/1(egrqcohbl) -> MinMax/2, Switch13/1, MinMax1/1
  egrtgstdly/1 -> AEMS_TIMER1/2, AEMS_TIMER2/2, AEMS_TIMER3/2, AEMS_TIMER4/2, AEMS_TIMER5/2, AEMS_TIMER/2, M2002_2A_2A_0x_EGR_DELAY_NR_10ms/2(egrtgstdly)  "egrtgstdly"
  Multiport Switch/1 -> M2002_2A_2A_0x_EGR_DELAY_NR_10ms/1(vegrqcohx_nr0)  "vegrqcohx_nr0"
  Switch9/1 -> Switch13/3, Unit Delay3/1  "egrqcoh_0"
  Unit Delay3/1 -> MinMax1/2, MinMax/1  "egrqcoh_z"
  MinMax1/1 -> Switch9/1
  MinMax/1 -> Switch9/3
  AEMS_EDGE_EITHER/1 -> Switch3/2, Logical Operator6/1, Logical Operator7/1, Logical Operator2/2, Logical Operator3/2, Logical Operator5/2, Logical Operator4/1, Switch1/2  "clear_set"
  Switch1/1 -> Relational Operator7/2, Switch7/3  "add1"
  Unit Delay1/1 -> Switch1/3, Sum2/2  "count1_pudt"
  Constant28/1 -> Relational Operator7/1
  Constant29/1 -> Switch7/1
  Relational Operator7/1 -> Switch7/2
  Switch7/1 -> Relational Operator14/1, Unit Delay1/1, Relational Operator10/1, Relational Operator4/1, Relational Operator5/1, Relational Operator3/1, Relational Operator1/1  "count1"
  Constant33/1 -> Sum2/1
  Sum2/1 -> Switch1/1
  Multiport Switch1/1 -> fegrqincx/1, Switch3/1, AEMS_EDGE_EITHER/1  "fegrqincx"
  Relational Operator14/1 -> Switch2/2, Logical Operator4/2  "and1"
  Constant22/1 -> Relational Operator14/2
  Constant23/1 -> Relational Operator10/2
  Relational Operator10/1 -> Switch4/2, Logical Operator6/2  "and2"
  Constant24/1 -> Relational Operator1/2
  Relational Operator1/1 -> Switch6/2, Logical Operator7/2  "and3"
  AEMS_TIMER/2 -> Terminator3/1
  AEMS_TIMER1/2 -> Terminator4/1
  AEMS_SRFLIPFLOP/1 -> AEMS_TIMER/1  "start_flag"
  Logical Operator4/1 -> AEMS_SRFLIPFLOP/1  "set"
  AEMS_SRFLIPFLOP1/1 -> AEMS_TIMER1/1  "start_flag"
  Logical Operator6/1 -> AEMS_SRFLIPFLOP1/1  "set"
  AEMS_SRFLIPFLOP2/1 -> AEMS_TIMER2/1  "start_flag"
  Logical Operator7/1 -> AEMS_SRFLIPFLOP2/1  "set"
  AEMS_TIMER2/2 -> Terminator1/1
  AEMS_TIMER/1 -> Unit Delay13/1, Logical Operator1/1
  AEMS_TIMER1/1 -> Unit Delay12/1, Logical Operator1/2
  AEMS_TIMER2/1 -> Unit Delay4/1, Logical Operator1/3
  Switch5/1 -> Switch8/3, Relational Operator2/2  "add"
  Unit Delay7/1 -> Sum/2, Switch5/3  "egrstcount_pudt"
  Constant12/1 -> Relational Operator2/1
  Relational Operator2/1 -> Switch8/2
  Switch8/1 -> Unit Delay7/1, Sum3/1  "count2"
  Constant13/1 -> Switch8/1
  Logical Operator1/1 -> Switch5/2
  Constant11/1 -> Sum/1
  Sum/1 -> Switch5/1
  Unit Delay6/1 -> Switch2/3
  Switch2/1 -> Unit Delay6/1, Multiport Switch2/3  "hold1"
  Unit Delay8/1 -> Switch4/3
  Switch4/1 -> Unit Delay8/1, Multiport Switch2/4  "hold2"
  Unit Delay9/1 -> Switch6/3
  Switch3/1 -> Switch2/1, Unit Delay10/1, Switch4/1, Switch6/1, Switch10/1, Switch11/1, Switch12/1  "temp"
  Unit Delay10/1 -> Switch3/3
  Switch6/1 -> Unit Delay9/1, Multiport Switch2/5  "temp"
  Sum3/1 -> Saturation1/1
  Constant14/1 -> Sum3/2
  Saturation1/1 -> Multiport Switch2/1
  Constant1/1 -> Multiport Switch2/2
  Multiport Switch2/1 -> Switch9/2  "fegrqinc"
  fegrqinc1/1 -> Multiport Switch1/2  "fegrqinc1"
  fegrqinc2/1 -> Multiport Switch1/3  "fegrqinc2"
  fegrqinc3/1 -> Multiport Switch1/4  "fegrqinc3"
  fegrqinc4/1 -> Multiport Switch1/5  "fegrqinc4"
  fegrqinc5/1 -> Multiport Switch1/6  "fegrqinc5"
  fegrqinc6/1 -> Multiport Switch1/7  "fegrqinc6"
  fegrqinc7/1 -> Multiport Switch1/8  "fegrqinc7"
  fegrqinc8/1 -> Multiport Switch1/9  "fegrqinc8"
  fegrqinc9/1 -> Multiport Switch1/10  "fegrqinc9"
  Saturation3/1 -> Multiport Switch/1
  Saturation2/1 -> Multiport Switch1/1

== system AEMS_Standard_Library/SPECIFIC/AEMS_EGR_OFFSET_BLOCK_DIM8 ==
  vegrhos_offset : Inport
      settings: AttributesFormatString=<tsample=%<SampleTime>>
  knockfb : Inport  Port=2
      settings: AttributesFormatString=<tsample=%<SampleTime>>
  AEMS_EDGE_RISING : AEMS_Standard_Library/EDGE/AEMS_EDGE_RISING  Tag=[LIB]  init=false
      settings: AttributesFormatString=|
      | %<MaskType>
      | Initial Value : %<init>
  AEMS_SRFLIPFLOP : AEMS_Standard_Library/FLAG/AEMS_SRFLIPFLOP  Tag=[LIB]  init=false
      settings: AttributesFormatString=%<MaskType>\nInitial condition (state of Q): = %<init>
  Add4 : Sum  Inputs=-+  SaturateOnIntegerOverflow=on  InputSameDT=on
  Add5 : Sum  Inputs=+-  SaturateOnIntegerOverflow=on  InputSameDT=on
  Add6 : Sum  Inputs=+-  SaturateOnIntegerOverflow=on  InputSameDT=on
  Add9 : Sum  Inputs=-+  SaturateOnIntegerOverflow=on  InputSameDT=on
  Constant1 : Constant  Value=10  OutDataTypeStr=single
  Constant14 : Constant  Value=-0.00001  OutDataTypeStr=single
  Constant17 : Constant  Value=0.00001  OutDataTypeStr=single
  Constant{18..19,21..22} (4 alike) : Constant  Value=0  OutDataTypeStr=single
  Constant20 : Constant  Value=Cxx_egrhsofs  OutDataTypeStr=Inherit: Inherit via back propagation
  Logical Operator10 : Logic  Operator=NAND  Inputs=3  OutDataTypeStr=boolean
  Logical Operator9 : Logic  Operator=NOT  Inputs=1  OutDataTypeStr=boolean
  MinMax : MinMax  Inputs=2  SaturateOnIntegerOverflow=on  InputSameDT=on
  Relational Operator2 : RelationalOperator  Operator=<  OutDataTypeStr=boolean  RndMeth=Nearest  InputSameDT=on
  Relational Operator3 : RelationalOperator  Operator=<  OutDataTypeStr=boolean  RndMeth=Nearest  InputSameDT=on
  Relational Operator4 : RelationalOperator  Operator=>  OutDataTypeStr=boolean  RndMeth=Nearest  InputSameDT=on
  Relational Operator5 : RelationalOperator  Operator=<  OutDataTypeStr=boolean  RndMeth=Nearest  InputSameDT=on
  Switch{8..13} (6 alike) : Switch  Threshold=0.5  SaturateOnIntegerOverflow=on  InputSameDT=on
      settings: AttributesFormatString=<threshold=%<Threshold>>
  Unit Delay{2..3,5..7} (5 alike) : UnitDelay  SampleTime=-1
      settings: AttributesFormatString=<initial=%<X0>>
  knkfbegr : Outport
  wires:
  Constant1/1 -> MinMax/1
  Relational Operator3/1 -> Logical Operator10/3
  MinMax/1 -> Relational Operator3/1, Unit Delay7/1
  Constant22/1 -> Switch13/3
  Constant20/1 -> Relational Operator3/2
  Add9/1 -> Switch12/3
  Constant21/1 -> Switch12/1
  Switch13/1 -> Add9/1
  Unit Delay7/1 -> Add9/2
  Switch12/1 -> MinMax/2
  Logical Operator9/1 -> Switch8/2
  Constant18/1 -> Switch8/1
  Add4/1 -> Switch8/3, Relational Operator4/2
  Constant14/1 -> Relational Operator5/2
  AEMS_EDGE_RISING/1 -> AEMS_SRFLIPFLOP/1  "set"
  Relational Operator4/1 -> Logical Operator10/2
  Logical Operator10/1 -> AEMS_SRFLIPFLOP/2  "clear"
  Unit Delay2/1 -> Add4/2
  Relational Operator5/1 -> Switch13/2, Switch10/2, AEMS_EDGE_RISING/1, Logical Operator10/1
  AEMS_SRFLIPFLOP/1 -> Switch11/2, Logical Operator9/1
  Add5/1 -> Switch11/1, Switch13/1, Add4/1, Relational Operator5/1
  Switch8/1 -> Unit Delay2/1
  Add6/1 -> Relational Operator4/1
  Constant19/1 -> Switch11/3
  Switch11/1 -> knkfbegr/1
  Unit Delay6/1 -> Switch10/1
  Switch10/1 -> Unit Delay6/1, Add6/1
  Unit Delay5/1 -> Switch9/3
  Switch9/1 -> Unit Delay5/1, Add6/2
  Relational Operator2/1 -> Switch12/2, Switch9/2
  Constant17/1 -> Relational Operator2/2
  Unit Delay3/1 -> Add5/2
  vegrhos_offset/1 -> Add5/1, Unit Delay3/1, Relational Operator2/1
  knockfb/1 -> Switch10/3, Switch9/1

== system AEMS_Standard_Library/SPECIFIC/AEMS_EGR_RATE_TRANSPORTOR_LIB ==
  vol_flow_rate : Inport  OutDataTypeStr=single
  egr_rate_in : Inport  Port=2  OutDataTypeStr=single
  dlt_profile_in : Inport  Port=3  OutDataTypeStr=single
  block1_vol : Inport  Port=4  OutDataTypeStr=single
  block2_vol : Inport  Port=5  OutDataTypeStr=single
  block3_vol : Inport  Port=6  OutDataTypeStr=single
  block_selector : Inport  Port=7
  block_1_transport : Subsystem
  block_2_transport : Subsystem
  block_3_transport : Subsystem
  dlt_profile_output_selector : Subsystem
  egr_rate_output_selector : Subsystem
  egr_rate_out1 : Outport
  egr_rate_out2 : Outport  Port=2
  egr_rate_out3 : Outport  Port=3
  egr_rate_out : Outport  Port=4
  dlt_profile_out : Outport  Port=5
  wires:
  block_2_transport/1(egr_rate_out2) -> egr_rate_out2/1, egr_rate_output_selector/3(egr_rate_out2), block_3_transport/2(egr_rate_out2)
  block_2_transport/2(dlt_profile_out2) -> dlt_profile_output_selector/2(dlt_profile_out2), block_3_transport/3(dlt_profile_out2)
  vol_flow_rate/1 -> block_2_transport/1(vol_flow_rate), block_3_transport/1(vol_flow_rate), block_1_transport/1(vol_flow_rate)
  block2_vol/1 -> block_2_transport/4(block2_vol)
  block3_vol/1 -> block_3_transport/4(block3_vol)
  block_3_transport/2(dlt_profile_out3) -> dlt_profile_output_selector/1(dlt_profile_out3)
  block_3_transport/1(egr_rate_out3) -> egr_rate_out3/1, egr_rate_output_selector/4(egr_rate_out3)
  block_selector/1 -> egr_rate_output_selector/1(block_selector), dlt_profile_output_selector/4(block_selector)
  egr_rate_output_selector/1(egr_rate_out) -> egr_rate_out/1
  egr_rate_in/1 -> block_1_transport/2(egr_rate_in)
  dlt_profile_in/1 -> block_1_transport/3(dlt_profile_in)
  block1_vol/1 -> block_1_transport/4(block1_vol)
  block_1_transport/1(egr_rate_out1) -> egr_rate_output_selector/2(egr_rate_out1), egr_rate_out1/1, block_2_transport/2(egr_rate_out1)
  block_1_transport/2(dlt_profile_out1) -> dlt_profile_output_selector/3(dlt_profile_out1), block_2_transport/3(dlt_profile_out1)
  dlt_profile_output_selector/1(dlt_profile_out) -> dlt_profile_out/1
